simulink model "SB10_logic_done"  (R2024b)
settings: Solver=FixedStepDiscrete  StartTime=0.0  StopTime=60  FixedStep=0.05  RelTol=1e-3
settings Model: Creator=admin  LastModifiedBy=admin

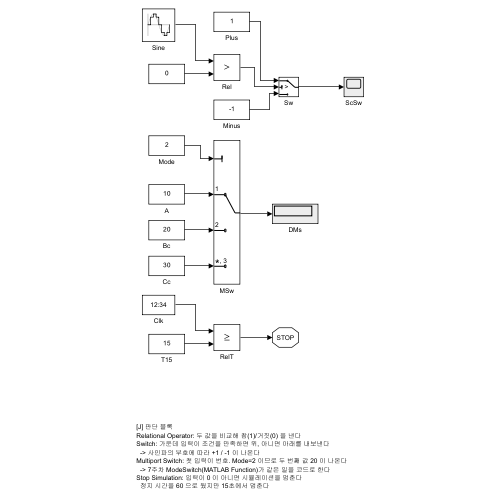
[thumbnail: Simulink's stored preview of the top-level diagram]
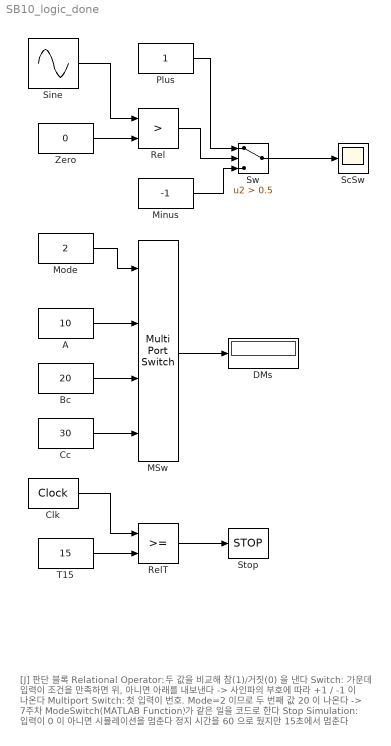
== system SB10_logic_done ==
  note: [J] 판단 블록
      | Relational Operator: 두 값을 비교해 참(1)/거짓(0) 을 낸다
      | Switch: 가운데 입력이 조건을 만족하면 위, 아니면 아래를 내보낸다
      |   -> 사인파의 부호에 따라 +1 / -1 이 나온다
      | Multiport Switch: 첫 입력이 번호. Mode=2 이므로 두 번째 값 20 이 나온다
      |   -> 7주차 ModeSwitch(MATLAB Function)가 같은 일을 코드로 한다
      | Stop Simulation: 입력이 0 이 아니면 시뮬레이션을 멈춘다
      |   정지 시간을 60 으로 뒀지만 15초에서 멈춘다
  A : Constant  Value=10
  Bc : Constant  Value=20
  Cc : Constant  Value=30
  Clk : DigitalClock  SampleTime=0.05
  DMs : Display
  MSw : MultiPortSwitch  SaturateOnIntegerOverflow=off  InputSameDT=off
  Minus : Constant  Value=-1
  Mode : Constant  Value=2
  Plus : Constant
  Rel : RelationalOperator  Operator=>  OutDataTypeStr=boolean  RndMeth=Simplest  InputSameDT=off
  RelT : RelationalOperator  OutDataTypeStr=boolean  RndMeth=Simplest  InputSameDT=off
  ScSw : Scope
  Sine : Sin  Frequency=0.5  SampleTime=0.05
  Stop : Stop
  Sw : Switch  Criteria=u2 > Threshold  Threshold=0.5  SaturateOnIntegerOverflow=off  InputSameDT=off
  T15 : Constant  Value=15
  Zero : Constant  Value=0
  wires:
  Sine/1 -> Rel/1
  Zero/1 -> Rel/2
  Cc/1 -> MSw/4
  Mode/1 -> MSw/1
  Bc/1 -> MSw/3
  Clk/1 -> RelT/1
  A/1 -> MSw/2
  T15/1 -> RelT/2
  Plus/1 -> Sw/1
  Rel/1 -> Sw/2
  Minus/1 -> Sw/3
  MSw/1 -> DMs/1
  RelT/1 -> Stop/1
  Sw/1 -> ScSw/1
